simulink model "ModeloMotorDC"  (R2013a)
settings: Solver=ode45  StartTime=0.0  StopTime=10.0  RelTol=1e-3
values from neighbouring files (symbols this model uses):
  Bd = 0.01979    [MotorDC.m]
  Bi = 0.01890    (= 0.0189)    [MotorDC.m]
  J = Je + Jr    (= 2.10171063337e-05)    [MotorDC.m]
  Kd = 0.2506    [MotorDC.m]
  Ki = 0.2530    (= 0.253)    [MotorDC.m]
  Ld = Td*(1+Rd)    (= 0.00030056)    [MotorDC.m]
  Li = Ti*(1+Ri)    (= 0.00025795)    [MotorDC.m]
  Rd = 1.312    [MotorDC.m]
  Ri = 1.345    [MotorDC.m]
  Va = 1.0    (= 1)    [MotorDC.m]
settings Model: Creator=user  LastModifiedBy=user

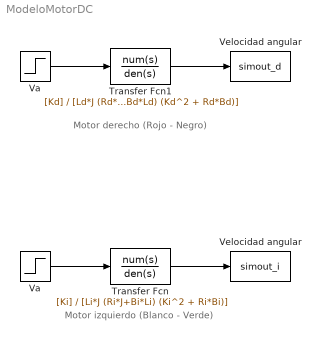
== system ModeloMotorDC ==
  note: Motor derecho (Rojo - Negro)
  note: Motor izquierdo (Blanco - Verde)
  Transfer Fcn : TransferFcn  Numerator=[Ki]  Denominator=[Li*J (Ri*J+Bi*Li) (Ki^2 + Ri*Bi)]
  Transfer Fcn1 : TransferFcn  Numerator=[Kd]  Denominator=[Ld*J (Rd*J+Bd*Ld) (Kd^2 + Rd*Bd)]
  Va : Step  After=Va  SampleTime=0
  "Va " : Step  After=Va  SampleTime=0
  Velocidad angular : ToWorkspace  VariableName=simout_d  SampleTime=-1  SaveFormat=Timeseries
  "Velocidad angular " : ToWorkspace  VariableName=simout_i  SampleTime=-1  SaveFormat=Timeseries
  wires:
  Va/1 -> Transfer Fcn/1
  Transfer Fcn/1 -> "Velocidad angular "/1
  "Va "/1 -> Transfer Fcn1/1
  Transfer Fcn1/1 -> Velocidad angular/1
